simulink model "mLarge_MajorAdjust_3"  (R2019a)
settings: Solver=ode45  StartTime=0  StopTime=2000  FixedStep=0.001  RelTol=1e-5  AbsTol=1e-6
PostLoadFcn:
  | sldemo_fuelsys_data(bdroot,'initialize_data','orig','float');
model workspace (MAT data in the model file):
  PressEst = [0.806253176324 0.553142316929 0.37151500209 0.277667903103 0.220198954207 0.181288665766 0.153200000489 0.115431020872 0.0913067476324 0.0746519188607 0.0625231108324 0.0533383634277 ... (306 elements, 18x17)]
  PressVect = [0.05 0.1 0.15 0.2 0.25 0.3 0.35 0.4 0.45 0.5 0.55 0.6 0.65 0.7 0.75 0.8 0.85 0.9 0.95]
  PumpCon = [-0.0556348 -0.0022828 0.0256932 0.0435188 0.0562692 0.0661194857143 0.0741572 0.08697 0.0972452 0.106070342857 0.1139892 0.121303866667 ... (342 elements, 18x19)]
  RampRateKiX = [100 200 300 400 500 600]
  RampRateKiY = [0 0.2 0.4 0.6 0.8 1]
  RampRateKiZ = [0.012  0.024  0.036  0.048  0.06  0.072; 0.024  0.048  0.072  0.096  0.12  0.144; 0.036  0.072  0.108  0.144  0.18  0.216; 0.048  0.096  0.144  0.192  0.24  0.288; 0.06  0.12  0.18  0.24  0.3  0.36; 0.072  0.144  0.216  0.288  0.36  0.432]
  SpeedEst = [471.837839721 550.80940091 777.559313277 1080.9243499 1418.36795322 1769.7468768 2125.37309264 2480.20345067 2831.37796793 3177.14006959 3516.32917143 4064.90417867 ... (323 elements, 17x19)]
  SpeedVect = [50 75 100 125 150 175 200 250 300 350 400 450 500 600 700 800 900 1000]
  ThrotEst = [0 0 0 0 0 0 0 0 0 0 0 0 ... (342 elements, 18x19)]
  ThrotVect = [0 3 6 9 12 15 18 21 24 27 30 35 46 57 68 79 90]
  ego_sw = 1
  engine_speed = 300
  hys = 25
  map_sw = 1
  max_ego = 1.2
  max_press = 0.95
  max_speed = 628
  max_throt = 90
  min_press = 0.05
  min_speed = 50
  min_throt = 3
  speed_sw = 1
  st_range = 0.0001
  throttle_sw = 1
  zero_thresh = 250
undefined symbols (not defined in the file): DiscIntNeverNeededParam, sld_FuelModes, sldvsubsys
libraries: simulink x16, simulink_extras x4
(part 1 of 3)
CloseFcn:
  | clear EngSensors u8En* s16En* sldemo_fuelsys_output
Description:
  | This is a model of a fuel control system where Stateflow(R) is used to handle the fault management of the system.
  | The system contains four separate sensors: a throttle sensor, a speed sensor, an oxygen sensor, and a pressure sensor.
  | Each of these sensors is represented by a parallel state in Stateflow.  Each parallel state contains two substates, a
  | normal state and a failed state (the exception being the oxygen sensor, which also contains a warmup state).
  | 
  | If any of the sensor readings is outside an acceptable range, then a fault is registered in Stateflow, and the
  | substate of the corresponding subsystem transitions to the failed state.  If a subsystem recovers, it can
  | transition back to the normal state.  The number of failures in the system at any given time is represented
  | in the Fail parallel state.
  | 
  | The last parallel state in the Stateflow chart is called Fueling_Mode.  This state regulates the oxygen to
  | fuel mixture ratio.  If a failure is detected, then the oxygen to fuel ratio is increased.  If multiple failures
  | are detected, then the fuel system is disabled until there are no longer multiple failures in the system.
settings Model: ModifiedByFormat=The MathWorks Inc.  ExtModeTrigMode=oneshot  ExtModeArmWhenConnect=off  ExtModeAutoUpdateStatusClock=off  Creator=The MathWorks, Inc.  LastModifiedBy=The MathWorks Inc.
settings SolverCC: AutoScaleAbsTol=off
settings DataIOCC: SaveFormat=StructureWithTime  SaveOutput=off  SaveTime=off  ReturnWorkspaceOutputs=off  SignalLoggingName=sldemo_fuelsys_output
settings OptimizationCC: DefaultParameterBehavior=Inlined  UseDivisionForNetSlopeComputation=UseDivisionForReciprocalsOfIntegersOnly  InlineInvariantSignals=on  EnhancedBackFolding=on  StrengthReduction=on  BooleansAsBitfields=on  PassReuseOutputArgsAs=Individual arguments  ExpressionDepthLimit=2147483647  ZeroExternalMemoryAtStartup=off  ZeroInternalMemoryAtStartup=off  NoFixptDivByZeroProtection=on  EfficientFloat2IntCast=on  LifeSpan=1
settings DebuggingCC: SignalInfNanChecking=error  SaveWithParameterizedLinksMsg=none  UnderspecifiedInitializationDetection=Classic  CheckExecutionContextPreStartOutputMsg=on  CheckExecutionContextRuntimeOutputMsg=on  IntegerOverflowMsg=none  ParameterDowncastMsg=warning  ParameterOverflowMsg=none  ParameterPrecisionLossMsg=none  UnderSpecifiedDataTypeMsg=warning  FcnCallInpInsideContextMsg=warning  UniqueDataStoreMsg=error  BusObjectLabelMismatch=error  AllowSymbolicDim=off  StateNameClashWarn=warning  StrictBusMsg=ErrorOnBusTreatedAsVector  SFUnexpectedBacktrackingDiag=warning  SFNoUnconditionalDefaultTransitionDiag=warning  SFExecutionAtInitializationDiag=none  IntegerSaturationMsg=none
settings HardwareCC: ProdBitPerPointer=32  ProdBitPerSizeT=32  ProdBitPerPtrDiffT=32  ProdLargestAtomicFloat=None  ProdWordSize=32  ProdHWDeviceType=Specified
settings ModelReferenceCC: PropagateSignalLabelsOutOfModel=off
settings SFSimCC: SimUseLocalCustomCode=off  SimParseCustomCode=off  MATLABDynamicMemAlloc=off
settings RTWCC: SystemTargetFile=ert.tlc  TemplateMakefile=ert_default_tmf  Description=Real-Time Workshop Embedded Coder  GenerateReport=on  RTWVerbose=off  RTWUseLocalCustomCode=off  IncludeHyperlinkInReport=on  LaunchReport=on  GenerateTraceInfo=on  GenerateTraceReport=on  GenerateTraceReportSl=on  GenerateTraceReportSf=on  GenerateTraceReportEml=on
settings CodeAppCC: ForceParamTrailComments=on  IgnoreCustomStorageClasses=off  IgnoreTestpoints=on  SimulinkDataObjDesc=on  SFDataObjDesc=on  CustomSymbolStrGlobalVar=rt$N$M  CustomSymbolStrType=$N$M  CustomSymbolStrFcn=$N$M$F  CustomSymbolStrModelFcn=$N  CustomSymbolStrMacro=$N$M  InsertBlockDesc=on  StateflowObjectComments=on  InternalIdentifier=Classic  ReqsInCode=on
settings ERTTargetCC: MultiwordLength=2048  GenerateSampleERTMain=on  IncludeMdlTerminateFcn=off  SupportAbsoluteTime=off  SupportNonFinite=off  SupportComplex=off  InlinedParameterPlacement=NonHierarchical  ERTCustomFileTemplate=example_file_process.tlc  ConvertIfToSwitch=off  SuppressUnreachableDefaultCases=off
settings ConfigComp: CovScope=Subsystem  CovPath=/fuel_rate_control/control_logic  CovMetricSettings=dw  CovHtmlReporting=on  CovSaveCumulativeToWorkspaceVar=on  CovSaveSingleToWorkspaceVar=on  CovShowResultsExplorer=off  CovExternalEMLEnable=off  CovSFcnEnable=off

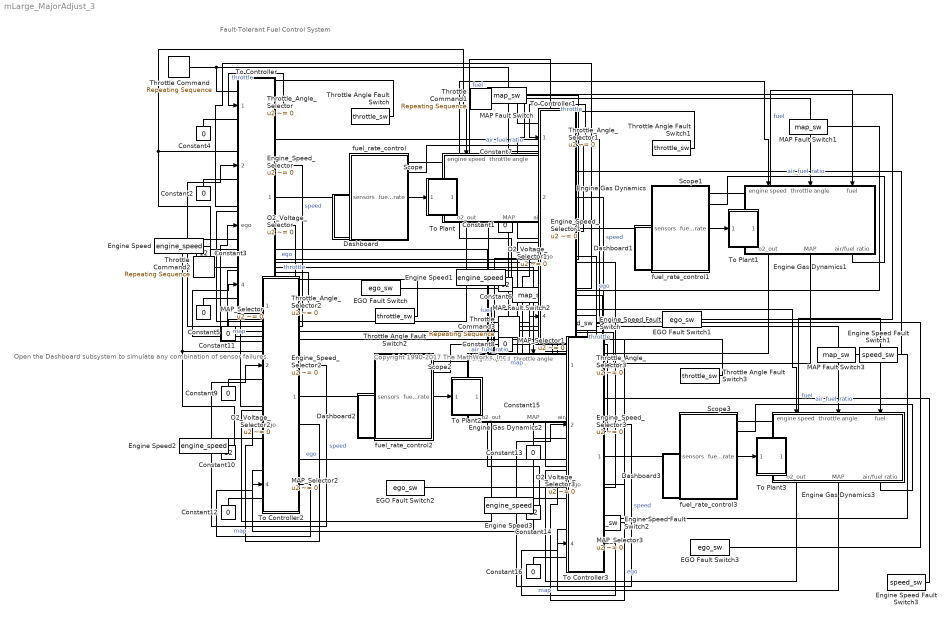
== system mLarge_MajorAdjust_3 ==
  note: Fault-Tolerant Fuel Control System
  note: Copyright 1990-2017 The MathWorks, Inc.
  note: Open the Dashboard subsystem to simulate any combination of sensor failures.
  Constant{1..2,4..5,7..9,11..13,15..16} (12 alike) : Constant  Value=0
  Constant{3,6,10,14} (4 alike) : Constant  Value=12
  Dashboard : Subsystem
  Dashboard1 : Subsystem
  Dashboard2 : Subsystem
  Dashboard3 : Subsystem
  EGO Fault Switch{,1..3} (4 alike) : Constant  Value=ego_sw
  Engine Gas Dynamics : Subsystem
  Engine Gas Dynamics1 : Subsystem
  Engine Gas Dynamics2 : Subsystem
  Engine Gas Dynamics3 : Subsystem
  Engine Speed{,1..3} (4 alike) : Constant  Value=engine_speed  SampleTime=[0,1]
  Engine Speed Fault Switch{,1..3} (4 alike) : Constant  Value=speed_sw
  Engine_Speed_Selector{,1..3} (4 alike) : Switch  Criteria=u2 ~= 0  Threshold=1
  MAP Fault Switch{,1..3} (4 alike) : Constant  Value=map_sw
  MAP_Selector{,1..3} (4 alike) : Switch  Criteria=u2 ~= 0  Threshold=1
  O2_Voltage_Selector{,1..3} (4 alike) : Switch  Criteria=u2 ~= 0  Threshold=1
  Scope{,1..3} (4 alike) : Scope  NumInputPorts=2
  Throttle Command{,1..3} (4 alike) : simulink/Sources/Repeating Sequence  rep_seq_t=[0 2 4]  rep_seq_y=[10 20 10]
  Throttle Angle Fault Switch{,1..3} (4 alike) : Constant  Value=throttle_sw
  Throttle_Angle_Selector{,1..3} (4 alike) : Switch  Criteria=u2 ~= 0  Threshold=1
  To Controller : Subsystem
      mask Display: fprintf('Convert')
  To Controller1 : Subsystem
      mask Display: fprintf('Convert')
  To Controller2 : Subsystem
      mask Display: fprintf('Convert')
  To Controller3 : Subsystem
      mask Display: fprintf('Convert')
  To Plant : Subsystem
      mask Display: fprintf('Convert')
  To Plant1 : Subsystem
      mask Display: fprintf('Convert')
  To Plant2 : Subsystem
      mask Display: fprintf('Convert')
  To Plant3 : Subsystem
      mask Display: fprintf('Convert')
  fuel_rate_control : Subsystem  Tag=FuelRateControl  TreatAsAtomicUnit=on
  fuel_rate_control1 : Subsystem  Tag=FuelRateControl  TreatAsAtomicUnit=on
  fuel_rate_control2 : Subsystem  Tag=FuelRateControl  TreatAsAtomicUnit=on
  fuel_rate_control3 : Subsystem  Tag=FuelRateControl  TreatAsAtomicUnit=on
  wires:
  fuel_rate_control/1(fuel_rate) -> To Plant/1(In1)
  To Plant/1(Out1) -> Scope/1, Engine Gas Dynamics/3(fuel)  "fuel"
  To Controller/1(sensors) -> fuel_rate_control/1(sensors)
  Throttle_Angle_Selector/1 -> To Controller/1(throttle)  "throttle"
  Engine_Speed_Selector/1 -> To Controller/2(speed)  "speed"
  O2_Voltage_Selector/1 -> To Controller/3(ego)  "ego"
  MAP_Selector/1 -> To Controller/4(map)  "map"
  Constant4/1 -> Throttle_Angle_Selector/3
  Throttle Command/1 -> Throttle_Angle_Selector/1, Engine Gas Dynamics/2(throttle angle)
  Throttle Angle Fault Switch/1 -> Throttle_Angle_Selector/2
  Engine Speed Fault Switch/1 -> Engine_Speed_Selector/2
  Engine Speed/1 -> Engine_Speed_Selector/1, Engine Gas Dynamics/1(engine speed)
  Constant2/1 -> Engine_Speed_Selector/3
  Constant3/1 -> O2_Voltage_Selector/3
  Engine Gas Dynamics/1(o2_out) -> O2_Voltage_Selector/1
  EGO Fault Switch/1 -> O2_Voltage_Selector/2
  MAP Fault Switch/1 -> MAP_Selector/2
  Engine Gas Dynamics/2(MAP) -> MAP_Selector/1
  Constant5/1 -> MAP_Selector/3
  Engine Gas Dynamics/3(air/fuel ratio) -> Scope/2  "air_fuel_ratio"
  Engine Speed Fault Switch1/1 -> Engine_Speed_Selector1/2
  fuel_rate_control1/1(fuel_rate) -> To Plant1/1(In1)
  O2_Voltage_Selector1/1 -> To Controller1/3(ego)  "ego"
  Engine Gas Dynamics1/3(air/fuel ratio) -> Scope1/2  "air_fuel_ratio"
  Throttle Angle Fault Switch1/1 -> Throttle_Angle_Selector1/2
  To Controller1/1(sensors) -> fuel_rate_control1/1(sensors)
  To Plant1/1(Out1) -> Scope1/1, Engine Gas Dynamics1/3(fuel)  "fuel"
  Engine_Speed_Selector1/1 -> To Controller1/2(speed)  "speed"
  Engine Gas Dynamics1/2(MAP) -> MAP_Selector1/1
  Constant8/1 -> MAP_Selector1/3
  MAP_Selector1/1 -> To Controller1/4(map)  "map"
  Constant7/1 -> Throttle_Angle_Selector1/3
  Throttle Command1/1 -> Throttle_Angle_Selector1/1, Engine Gas Dynamics1/2(throttle angle)
  Constant6/1 -> O2_Voltage_Selector1/3
  Engine Speed1/1 -> Engine_Speed_Selector1/1, Engine Gas Dynamics1/1(engine speed)
  Throttle_Angle_Selector1/1 -> To Controller1/1(throttle)  "throttle"
  MAP Fault Switch1/1 -> MAP_Selector1/2
  Engine Gas Dynamics1/1(o2_out) -> O2_Voltage_Selector1/1
  EGO Fault Switch1/1 -> O2_Voltage_Selector1/2
  Constant1/1 -> Engine_Speed_Selector1/3
  Engine Speed Fault Switch2/1 -> Engine_Speed_Selector2/2
  fuel_rate_control2/1(fuel_rate) -> To Plant2/1(In1)
  O2_Voltage_Selector2/1 -> To Controller2/3(ego)  "ego"
  Engine Gas Dynamics2/3(air/fuel ratio) -> Scope2/2  "air_fuel_ratio"
  Throttle Angle Fault Switch2/1 -> Throttle_Angle_Selector2/2
  To Controller2/1(sensors) -> fuel_rate_control2/1(sensors)
  To Plant2/1(Out1) -> Scope2/1, Engine Gas Dynamics2/3(fuel)  "fuel"
  Engine_Speed_Selector2/1 -> To Controller2/2(speed)  "speed"
  Engine Gas Dynamics2/2(MAP) -> MAP_Selector2/1
  Constant12/1 -> MAP_Selector2/3
  MAP_Selector2/1 -> To Controller2/4(map)  "map"
  Constant11/1 -> Throttle_Angle_Selector2/3
  Throttle Command2/1 -> Throttle_Angle_Selector2/1, Engine Gas Dynamics2/2(throttle angle)
  Constant10/1 -> O2_Voltage_Selector2/3
  Engine Speed2/1 -> Engine_Speed_Selector2/1, Engine Gas Dynamics2/1(engine speed)
  Throttle_Angle_Selector2/1 -> To Controller2/1(throttle)  "throttle"
  MAP Fault Switch2/1 -> MAP_Selector2/2
  Engine Gas Dynamics2/1(o2_out) -> O2_Voltage_Selector2/1
  EGO Fault Switch2/1 -> O2_Voltage_Selector2/2
  Constant9/1 -> Engine_Speed_Selector2/3
  Engine Speed Fault Switch3/1 -> Engine_Speed_Selector3/2
  fuel_rate_control3/1(fuel_rate) -> To Plant3/1(In1)
  O2_Voltage_Selector3/1 -> To Controller3/3(ego)  "ego"
  Engine Gas Dynamics3/3(air/fuel ratio) -> Scope3/2  "air_fuel_ratio"
  Throttle Angle Fault Switch3/1 -> Throttle_Angle_Selector3/2
  To Controller3/1(sensors) -> fuel_rate_control3/1(sensors)
  To Plant3/1(Out1) -> Scope3/1, Engine Gas Dynamics3/3(fuel)  "fuel"
  Engine_Speed_Selector3/1 -> To Controller3/2(speed)  "speed"
  Engine Gas Dynamics3/2(MAP) -> MAP_Selector3/1
  Constant16/1 -> MAP_Selector3/3
  MAP_Selector3/1 -> To Controller3/4(map)  "map"
  Constant15/1 -> Throttle_Angle_Selector3/3
  Throttle Command3/1 -> Throttle_Angle_Selector3/1, Engine Gas Dynamics3/2(throttle angle)
  Constant14/1 -> O2_Voltage_Selector3/3
  Engine Speed3/1 -> Engine_Speed_Selector3/1, Engine Gas Dynamics3/1(engine speed)
  Throttle_Angle_Selector3/1 -> To Controller3/1(throttle)  "throttle"
  MAP Fault Switch3/1 -> MAP_Selector3/2
  Engine Gas Dynamics3/1(o2_out) -> O2_Voltage_Selector3/1
  EGO Fault Switch3/1 -> O2_Voltage_Selector3/2
  Constant13/1 -> Engine_Speed_Selector3/3

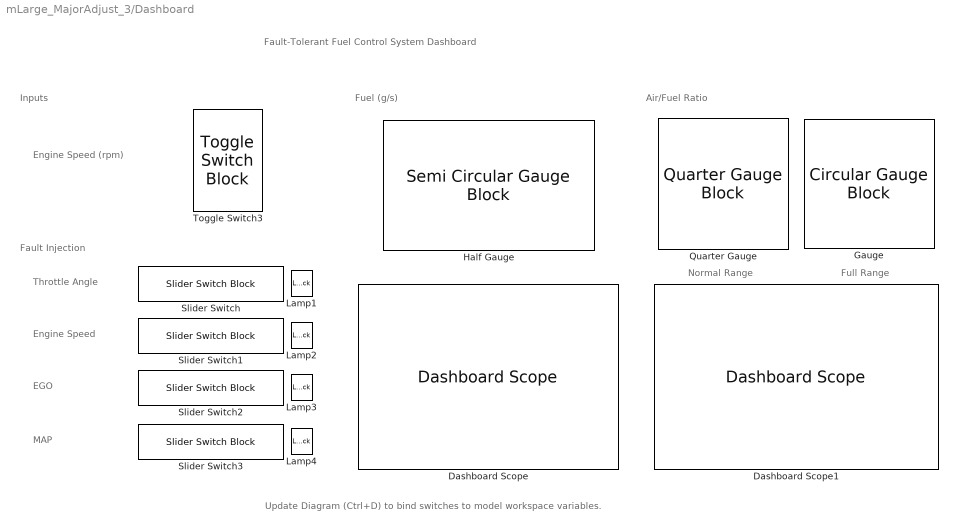
== system mLarge_MajorAdjust_3/Dashboard ==
  note: Inputs
  note: Fault Injection
  note: Air/Fuel Ratio
  note: Fuel (g/s)
  note: Throttle Angle
  note: Engine Speed
  note: EGO
  note: Fault-Tolerant Fuel Control System Dashboard
  note: MAP
  note: Engine Speed (rpm)
  note: Normal Range
  note: Full Range
  note: Update Diagram (Ctrl+D) to bind switches to model workspace variables.
  Dashboard Scope : DashboardScope  WebBlockId=348  TimeSpan=500  Ymin=0  LegendPosition=Hide  ScaleAtStop=off
  Dashboard Scope1 : DashboardScope  WebBlockId=349  TimeSpan=500  Ymin=0  Ymax=400  LegendPosition=Hide  ScaleAtStop=off
  Gauge : CircularGaugeBlock  WebBlockId=346  LabelPosition=Hide  ScaleMax=400
  Half Gauge : SemiCircularGaugeBlock  WebBlockId=347  LabelPosition=Hide  ScaleMax=3
  Lamp1 : LampBlock  WebBlockId=337  LabelPosition=Hide
  Lamp2 : LampBlock  WebBlockId=338  LabelPosition=Hide
  Lamp3 : LampBlock  WebBlockId=343  LabelPosition=Hide
  Lamp4 : LampBlock  WebBlockId=339  LabelPosition=Hide
  Quarter Gauge : QuarterGaugeBlock  WebBlockId=345  LabelPosition=Hide  ScaleMax=20
  Slider Switch : SliderSwitchBlock  WebBlockId=341  LabelPosition=Hide
      settings: Values={{'NORMAL', 'FAIL'}, [1 0]}
  Slider Switch1 : SliderSwitchBlock  WebBlockId=342  LabelPosition=Hide
      settings: Values={{'NORMAL', 'FAIL'}, [1 0]}
  Slider Switch2 : SliderSwitchBlock  WebBlockId=344  LabelPosition=Hide
      settings: Values={{'NORMAL', 'FAIL'}, [1 0]}
  Slider Switch3 : SliderSwitchBlock  WebBlockId=340  LabelPosition=Hide
      settings: Values={{'NORMAL', 'FAIL'}, [1 0]}
  Toggle Switch3 : ToggleSwitchBlock  WebBlockId=336  LabelPosition=Hide
      settings: Values={{'700', '300'}, [700 300]}

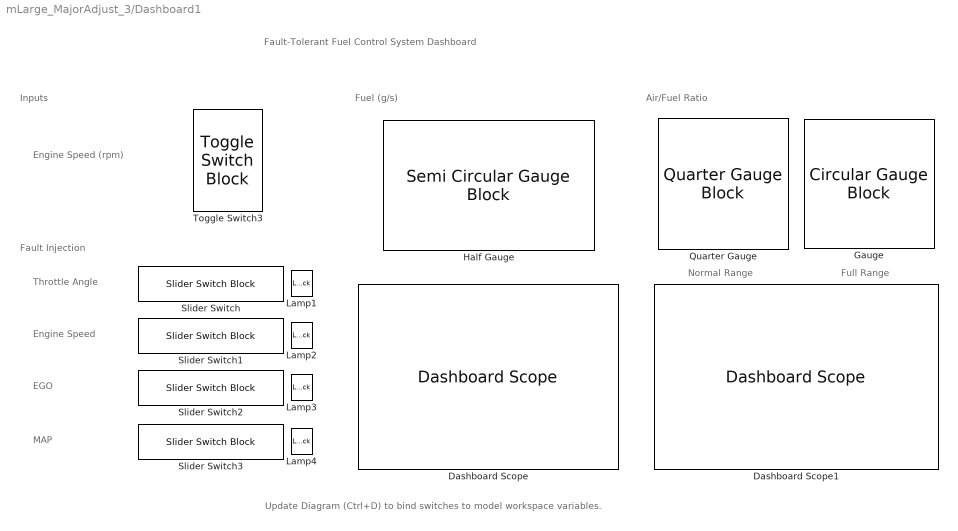
== system mLarge_MajorAdjust_3/Dashboard1 ==
  note: Inputs
  note: Fault Injection
  note: Air/Fuel Ratio
  note: Fuel (g/s)
  note: Throttle Angle
  note: Engine Speed
  note: EGO
  note: Fault-Tolerant Fuel Control System Dashboard
  note: MAP
  note: Engine Speed (rpm)
  note: Normal Range
  note: Full Range
  note: Update Diagram (Ctrl+D) to bind switches to model workspace variables.
  Dashboard Scope : DashboardScope  WebBlockId=355  TimeSpan=500  Ymin=0  LegendPosition=Hide  ScaleAtStop=off
  Dashboard Scope1 : DashboardScope  WebBlockId=356  TimeSpan=500  Ymin=0  Ymax=400  LegendPosition=Hide  ScaleAtStop=off
  Gauge : CircularGaugeBlock  WebBlockId=357  LabelPosition=Hide  ScaleMax=400
  Half Gauge : SemiCircularGaugeBlock  WebBlockId=358  LabelPosition=Hide  ScaleMax=3
  Lamp1 : LampBlock  WebBlockId=359  LabelPosition=Hide
  Lamp2 : LampBlock  WebBlockId=360  LabelPosition=Hide
  Lamp3 : LampBlock  WebBlockId=361  LabelPosition=Hide
  Lamp4 : LampBlock  WebBlockId=362  LabelPosition=Hide
  Quarter Gauge : QuarterGaugeBlock  WebBlockId=363  LabelPosition=Hide  ScaleMax=20
  Slider Switch : SliderSwitchBlock  WebBlockId=364  LabelPosition=Hide
      settings: Values={{'NORMAL', 'FAIL'}, [1 0]}
  Slider Switch1 : SliderSwitchBlock  WebBlockId=365  LabelPosition=Hide
      settings: Values={{'NORMAL', 'FAIL'}, [1 0]}
  Slider Switch2 : SliderSwitchBlock  WebBlockId=366  LabelPosition=Hide
      settings: Values={{'NORMAL', 'FAIL'}, [1 0]}
  Slider Switch3 : SliderSwitchBlock  WebBlockId=367  LabelPosition=Hide
      settings: Values={{'NORMAL', 'FAIL'}, [1 0]}
  Toggle Switch3 : ToggleSwitchBlock  WebBlockId=368  LabelPosition=Hide
      settings: Values={{'700', '300'}, [700 300]}

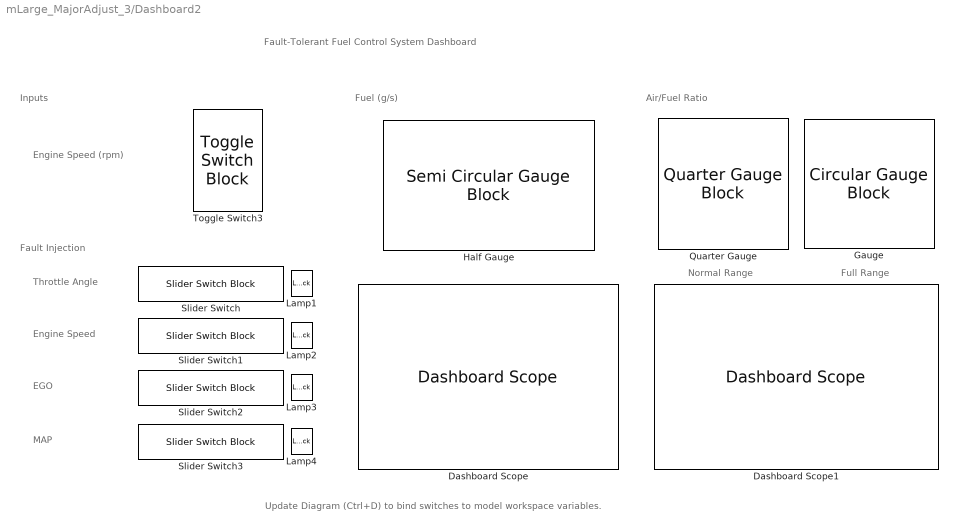
== system mLarge_MajorAdjust_3/Dashboard2 ==
  note: Inputs
  note: Fault Injection
  note: Air/Fuel Ratio
  note: Fuel (g/s)
  note: Throttle Angle
  note: Engine Speed
  note: EGO
  note: Fault-Tolerant Fuel Control System Dashboard
  note: MAP
  note: Engine Speed (rpm)
  note: Normal Range
  note: Full Range
  note: Update Diagram (Ctrl+D) to bind switches to model workspace variables.
  Dashboard Scope : DashboardScope  WebBlockId=551  TimeSpan=500  Ymin=0  LegendPosition=Hide  ScaleAtStop=off
  Dashboard Scope1 : DashboardScope  WebBlockId=552  TimeSpan=500  Ymin=0  Ymax=400  LegendPosition=Hide  ScaleAtStop=off
  Gauge : CircularGaugeBlock  WebBlockId=553  LabelPosition=Hide  ScaleMax=400
  Half Gauge : SemiCircularGaugeBlock  WebBlockId=554  LabelPosition=Hide  ScaleMax=3
  Lamp1 : LampBlock  WebBlockId=555  LabelPosition=Hide
  Lamp2 : LampBlock  WebBlockId=556  LabelPosition=Hide
  Lamp3 : LampBlock  WebBlockId=557  LabelPosition=Hide
  Lamp4 : LampBlock  WebBlockId=558  LabelPosition=Hide
  Quarter Gauge : QuarterGaugeBlock  WebBlockId=559  LabelPosition=Hide  ScaleMax=20
  Slider Switch : SliderSwitchBlock  WebBlockId=560  LabelPosition=Hide
      settings: Values={{'NORMAL', 'FAIL'}, [1 0]}
  Slider Switch1 : SliderSwitchBlock  WebBlockId=561  LabelPosition=Hide
      settings: Values={{'NORMAL', 'FAIL'}, [1 0]}
  Slider Switch2 : SliderSwitchBlock  WebBlockId=562  LabelPosition=Hide
      settings: Values={{'NORMAL', 'FAIL'}, [1 0]}
  Slider Switch3 : SliderSwitchBlock  WebBlockId=563  LabelPosition=Hide
      settings: Values={{'NORMAL', 'FAIL'}, [1 0]}
  Toggle Switch3 : ToggleSwitchBlock  WebBlockId=564  LabelPosition=Hide
      settings: Values={{'700', '300'}, [700 300]}

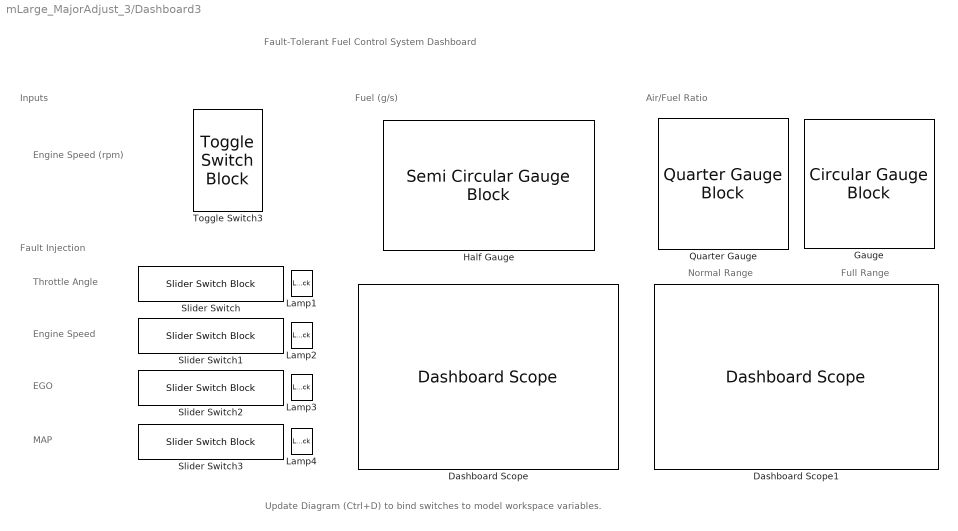
== system mLarge_MajorAdjust_3/Dashboard3 ==
  note: Inputs
  note: Fault Injection
  note: Air/Fuel Ratio
  note: Fuel (g/s)
  note: Throttle Angle
  note: Engine Speed
  note: EGO
  note: Fault-Tolerant Fuel Control System Dashboard
  note: MAP
  note: Engine Speed (rpm)
  note: Normal Range
  note: Full Range
  note: Update Diagram (Ctrl+D) to bind switches to model workspace variables.
  Dashboard Scope : DashboardScope  WebBlockId=747  TimeSpan=500  Ymin=0  LegendPosition=Hide  ScaleAtStop=off
  Dashboard Scope1 : DashboardScope  WebBlockId=748  TimeSpan=500  Ymin=0  Ymax=400  LegendPosition=Hide  ScaleAtStop=off
  Gauge : CircularGaugeBlock  WebBlockId=749  LabelPosition=Hide  ScaleMax=400
  Half Gauge : SemiCircularGaugeBlock  WebBlockId=750  LabelPosition=Hide  ScaleMax=3
  Lamp1 : LampBlock  WebBlockId=751  LabelPosition=Hide
  Lamp2 : LampBlock  WebBlockId=752  LabelPosition=Hide
  Lamp3 : LampBlock  WebBlockId=753  LabelPosition=Hide
  Lamp4 : LampBlock  WebBlockId=754  LabelPosition=Hide
  Quarter Gauge : QuarterGaugeBlock  WebBlockId=755  LabelPosition=Hide  ScaleMax=20
  Slider Switch : SliderSwitchBlock  WebBlockId=756  LabelPosition=Hide
      settings: Values={{'NORMAL', 'FAIL'}, [1 0]}
  Slider Switch1 : SliderSwitchBlock  WebBlockId=757  LabelPosition=Hide
      settings: Values={{'NORMAL', 'FAIL'}, [1 0]}
  Slider Switch2 : SliderSwitchBlock  WebBlockId=758  LabelPosition=Hide
      settings: Values={{'NORMAL', 'FAIL'}, [1 0]}
  Slider Switch3 : SliderSwitchBlock  WebBlockId=759  LabelPosition=Hide
      settings: Values={{'NORMAL', 'FAIL'}, [1 0]}
  Toggle Switch3 : ToggleSwitchBlock  WebBlockId=760  LabelPosition=Hide
      settings: Values={{'700', '300'}, [700 300]}

== system mLarge_MajorAdjust_3/Engine Gas Dynamics ==
  engine speed : Inport  Unit=rad/s
  throttle angle : Inport  Port=2  Unit=deg
  fuel : Inport  Port=3  Unit=g/s
  Mixing & Combustion : Subsystem
  Throttle & Manifold : Subsystem
  o2_out : Outport  Unit=V
  MAP : Outport  Port=2  Unit=bar
  air/fuel ratio : Outport  Port=3  Unit=1
  wires:
  Throttle & Manifold/1(Mass Airflow Rate) -> Mixing & Combustion/2(air flow)
  fuel/1 -> Mixing & Combustion/1(fuel rate)
  engine speed/1 -> Throttle & Manifold/1("Engine Speed, N")
  throttle angle/1 -> Throttle & Manifold/2(Throttle Ang.)
  Mixing & Combustion/2(air/fuel ratio) -> air/fuel ratio/1
  Throttle & Manifold/2(MAP (bar)) -> MAP/1
  Mixing & Combustion/1(o2_out) -> o2_out/1

== system mLarge_MajorAdjust_3/Engine Gas Dynamics1 ==
  engine speed : Inport  Unit=rad/s
  throttle angle : Inport  Port=2  Unit=deg
  fuel : Inport  Port=3  Unit=g/s
  Mixing & Combustion : Subsystem
  Throttle & Manifold : Subsystem
  o2_out : Outport  Unit=V
  MAP : Outport  Port=2  Unit=bar
  air/fuel ratio : Outport  Port=3  Unit=1
  wires:
  Throttle & Manifold/1(Mass Airflow Rate) -> Mixing & Combustion/2(air flow)
  fuel/1 -> Mixing & Combustion/1(fuel rate)
  engine speed/1 -> Throttle & Manifold/1("Engine Speed, N")
  throttle angle/1 -> Throttle & Manifold/2(Throttle Ang.)
  Mixing & Combustion/2(air/fuel ratio) -> air/fuel ratio/1
  Throttle & Manifold/2(MAP (bar)) -> MAP/1
  Mixing & Combustion/1(o2_out) -> o2_out/1

== system mLarge_MajorAdjust_3/Engine Gas Dynamics2 ==
  engine speed : Inport  Unit=rad/s
  throttle angle : Inport  Port=2  Unit=deg
  fuel : Inport  Port=3  Unit=g/s
  Mixing & Combustion : Subsystem
  Throttle & Manifold : Subsystem
  o2_out : Outport  Unit=V
  MAP : Outport  Port=2  Unit=bar
  air/fuel ratio : Outport  Port=3  Unit=1
  wires:
  Throttle & Manifold/1(Mass Airflow Rate) -> Mixing & Combustion/2(air flow)
  fuel/1 -> Mixing & Combustion/1(fuel rate)
  engine speed/1 -> Throttle & Manifold/1("Engine Speed, N")
  throttle angle/1 -> Throttle & Manifold/2(Throttle Ang.)
  Mixing & Combustion/2(air/fuel ratio) -> air/fuel ratio/1
  Throttle & Manifold/2(MAP (bar)) -> MAP/1
  Mixing & Combustion/1(o2_out) -> o2_out/1

== system mLarge_MajorAdjust_3/Engine Gas Dynamics3 ==
  engine speed : Inport  Unit=rad/s
  throttle angle : Inport  Port=2  Unit=deg
  fuel : Inport  Port=3  Unit=g/s
  Mixing & Combustion : Subsystem
  Throttle & Manifold : Subsystem
  o2_out : Outport  Unit=V
  MAP : Outport  Port=2  Unit=bar
  air/fuel ratio : Outport  Port=3  Unit=1
  wires:
  Throttle & Manifold/1(Mass Airflow Rate) -> Mixing & Combustion/2(air flow)
  fuel/1 -> Mixing & Combustion/1(fuel rate)
  engine speed/1 -> Throttle & Manifold/1("Engine Speed, N")
  throttle angle/1 -> Throttle & Manifold/2(Throttle Ang.)
  Mixing & Combustion/2(air/fuel ratio) -> air/fuel ratio/1
  Throttle & Manifold/2(MAP (bar)) -> MAP/1
  Mixing & Combustion/1(o2_out) -> o2_out/1

== system mLarge_MajorAdjust_3/To Controller ==
  note: This system:
      | - Packs individual sensors into a EngSensors bus signal
      | - Permits bus elements data types to change
      | - Converts signals from continuous to discrete time
  throttle : Inport
  speed : Inport  Port=2
  ego : Inport  Port=3
  map : Inport  Port=4
  Bus Creator : BusCreator  Inputs=4  OutDataTypeStr=Bus: EngSensors  NonVirtualBus=on
  DTC{1..4} (4 alike) : DataTypeConversion  SampleTime=[0 1]
  Rate Transition : RateTransition  OutPortSampleTime=0.01
  Sensor Info : simulink/Model-Wide Utilities/DocBlock  DocumentType=Text
      content=|
      | Measurement Descriptions
      | ========================
      |
      | Throttle Angle (degrees):
      | min=3, max=90, precision=0.1
      |
      | Engine Speed (radians/sec.):
      | min=0, max=620, precision=.1
      |
      | Ego Sensor (volts):
      | min=0, max=12, precision=.05
      |
      | Manifold Pressure (bar):
      | min=0.001, max=1, precision=.001
  sensors : Outport
  wires:
  throttle/1 -> DTC1/1
  DTC1/1 -> Bus Creator/1  "throttle"
  speed/1 -> DTC2/1
  DTC2/1 -> Bus Creator/2  "speed"
  ego/1 -> DTC3/1
  DTC3/1 -> Bus Creator/3  "ego"
  map/1 -> DTC4/1
  DTC4/1 -> Bus Creator/4  "map"
  Bus Creator/1 -> Rate Transition/1
  Rate Transition/1 -> sensors/1

== system mLarge_MajorAdjust_3/To Controller1 ==
  note: This system:
      | - Packs individual sensors into a EngSensors bus signal
      | - Permits bus elements data types to change
      | - Converts signals from continuous to discrete time
  throttle : Inport
  speed : Inport  Port=2
  ego : Inport  Port=3
  map : Inport  Port=4
  Bus Creator : BusCreator  Inputs=4  OutDataTypeStr=Bus: EngSensors  NonVirtualBus=on
  DTC{1..4} (4 alike) : DataTypeConversion  SampleTime=[0 1]
  Rate Transition : RateTransition  OutPortSampleTime=0.01
  Sensor Info : simulink/Model-Wide Utilities/DocBlock  DocumentType=Text
      content=|
      | Measurement Descriptions
      | ========================
      |
      | Throttle Angle (degrees):
      | min=3, max=90, precision=0.1
      |
      | Engine Speed (radians/sec.):
      | min=0, max=620, precision=.1
      |
      | Ego Sensor (volts):
      | min=0, max=12, precision=.05
      |
      | Manifold Pressure (bar):
      | min=0.001, max=1, precision=.001
  sensors : Outport
  wires:
  throttle/1 -> DTC1/1
  DTC1/1 -> Bus Creator/1  "throttle"
  speed/1 -> DTC2/1
  DTC2/1 -> Bus Creator/2  "speed"
  ego/1 -> DTC3/1
  DTC3/1 -> Bus Creator/3  "ego"
  map/1 -> DTC4/1
  DTC4/1 -> Bus Creator/4  "map"
  Bus Creator/1 -> Rate Transition/1
  Rate Transition/1 -> sensors/1

== system mLarge_MajorAdjust_3/To Controller2 ==
  note: This system:
      | - Packs individual sensors into a EngSensors bus signal
      | - Permits bus elements data types to change
      | - Converts signals from continuous to discrete time
  throttle : Inport
  speed : Inport  Port=2
  ego : Inport  Port=3
  map : Inport  Port=4
  Bus Creator : BusCreator  Inputs=4  OutDataTypeStr=Bus: EngSensors  NonVirtualBus=on
  DTC{1..4} (4 alike) : DataTypeConversion  SampleTime=[0 1]
  Rate Transition : RateTransition  OutPortSampleTime=0.01
  Sensor Info : simulink/Model-Wide Utilities/DocBlock  DocumentType=Text
      content=|
      | Measurement Descriptions
      | ========================
      |
      | Throttle Angle (degrees):
      | min=3, max=90, precision=0.1
      |
      | Engine Speed (radians/sec.):
      | min=0, max=620, precision=.1
      |
      | Ego Sensor (volts):
      | min=0, max=12, precision=.05
      |
      | Manifold Pressure (bar):
      | min=0.001, max=1, precision=.001
  sensors : Outport
  wires:
  throttle/1 -> DTC1/1
  DTC1/1 -> Bus Creator/1  "throttle"
  speed/1 -> DTC2/1
  DTC2/1 -> Bus Creator/2  "speed"
  ego/1 -> DTC3/1
  DTC3/1 -> Bus Creator/3  "ego"
  map/1 -> DTC4/1
  DTC4/1 -> Bus Creator/4  "map"
  Bus Creator/1 -> Rate Transition/1
  Rate Transition/1 -> sensors/1

== system mLarge_MajorAdjust_3/To Controller3 ==
  note: This system:
      | - Packs individual sensors into a EngSensors bus signal
      | - Permits bus elements data types to change
      | - Converts signals from continuous to discrete time
  throttle : Inport
  speed : Inport  Port=2
  ego : Inport  Port=3
  map : Inport  Port=4
  Bus Creator : BusCreator  Inputs=4  OutDataTypeStr=Bus: EngSensors  NonVirtualBus=on
  DTC{1..4} (4 alike) : DataTypeConversion  SampleTime=[0 1]
  Rate Transition : RateTransition  OutPortSampleTime=0.01
  Sensor Info : simulink/Model-Wide Utilities/DocBlock  DocumentType=Text
      content=|
      | Measurement Descriptions
      | ========================
      |
      | Throttle Angle (degrees):
      | min=3, max=90, precision=0.1
      |
      | Engine Speed (radians/sec.):
      | min=0, max=620, precision=.1
      |
      | Ego Sensor (volts):
      | min=0, max=12, precision=.05
      |
      | Manifold Pressure (bar):
      | min=0.001, max=1, precision=.001
  sensors : Outport
  wires:
  throttle/1 -> DTC1/1
  DTC1/1 -> Bus Creator/1  "throttle"
  speed/1 -> DTC2/1
  DTC2/1 -> Bus Creator/2  "speed"
  ego/1 -> DTC3/1
  DTC3/1 -> Bus Creator/3  "ego"
  map/1 -> DTC4/1
  DTC4/1 -> Bus Creator/4  "map"
  Bus Creator/1 -> Rate Transition/1
  Rate Transition/1 -> sensors/1

== system mLarge_MajorAdjust_3/To Plant ==
  note: This system:
      | - Permits upstream signal data type to change
      | - Converts signals from discrete to continuous time
  In1 : Inport
  DTC5 : DataTypeConversion
  Rate Transition1 : RateTransition  Integrity=off  InitialCondition=1.6  OutPortSampleTime=0
  Out1 : Outport
  wires:
  DTC5/1 -> Rate Transition1/1
  In1/1 -> DTC5/1
  Rate Transition1/1 -> Out1/1

== system mLarge_MajorAdjust_3/To Plant1 ==
  note: This system:
      | - Permits upstream signal data type to change
      | - Converts signals from discrete to continuous time
  In1 : Inport
  DTC5 : DataTypeConversion
  Rate Transition1 : RateTransition  Integrity=off  InitialCondition=1.6  OutPortSampleTime=0
  Out1 : Outport
  wires:
  DTC5/1 -> Rate Transition1/1
  In1/1 -> DTC5/1
  Rate Transition1/1 -> Out1/1

== system mLarge_MajorAdjust_3/To Plant2 ==
  note: This system:
      | - Permits upstream signal data type to change
      | - Converts signals from discrete to continuous time
  In1 : Inport
  DTC5 : DataTypeConversion
  Rate Transition1 : RateTransition  Integrity=off  InitialCondition=1.6  OutPortSampleTime=0
  Out1 : Outport
  wires:
  DTC5/1 -> Rate Transition1/1
  In1/1 -> DTC5/1
  Rate Transition1/1 -> Out1/1

== system mLarge_MajorAdjust_3/To Plant3 ==
  note: This system:
      | - Permits upstream signal data type to change
      | - Converts signals from discrete to continuous time
  In1 : Inport
  DTC5 : DataTypeConversion
  Rate Transition1 : RateTransition  Integrity=off  InitialCondition=1.6  OutPortSampleTime=0
  Out1 : Outport
  wires:
  DTC5/1 -> Rate Transition1/1
  In1/1 -> DTC5/1
  Rate Transition1/1 -> Out1/1

== system mLarge_MajorAdjust_3/fuel_rate_control ==
  note: Fuel Rate Control Subsystem
  sensors : Inport  OutDataTypeStr=Bus: EngSensors
  Bus Selector1 : BusSelector  OutputSignals=speed
  airflow_calc : Subsystem
  control_logic : Stateflow chart  Description=Stateflow diagram to determine control system operating mode  TreatAsAtomicUnit=on
  fuel_calc : Subsystem
  validate_sample_time : Subsystem  Tag=VerificationSubsystem  DisableCoverage=on  LoadFcn=sldvsubsys('check')  TreatAsAtomicUnit=on  SimViewingDevice=on  mask(VerificationSubsystem){}
      mask init:
      | sldvsubsys('maskInit');
      settings: CopyFcn=sldvsubsys('copy');  OpenFcn=open_system(gcb,'force');
      settings: PreSaveFcn=|
      | set_param(gcb,'SimViewingDevice','on');
      | sldvsubsys('check');
      mask Help: helpview(fullfile(docroot,'toolbox','sldv','sldv.map'),'verificationsubsystem')
      mask Display: image(imread('sldvicon_versubsys.png','BackGroundColor',[1 1 1]),'center');
  fuel_rate : Outport  Unit=g/s
  wires:
  fuel_calc/1(fuel_rate) -> fuel_rate/1
  airflow_calc/1(est_airflow) -> fuel_calc/1(est_airflow)
  sensors/1 -> control_logic/1(es_i), Bus Selector1/1
  control_logic/3(fuel_mode) -> airflow_calc/3(fuel_mode), fuel_calc/3(fuel_mode)
  control_logic/1(es_o) -> airflow_calc/1(sensors)
  control_logic/2(" O2_normal") -> airflow_calc/2(O2_normal)
  airflow_calc/2(fb_correction) -> fuel_calc/2(fb_correction)
  Bus Selector1/1 -> validate_sample_time/1(In1)  "<speed>"

== system mLarge_MajorAdjust_3/fuel_rate_control1 ==
  note: Fuel Rate Control Subsystem
  sensors : Inport  OutDataTypeStr=Bus: EngSensors
  Bus Selector1 : BusSelector  OutputSignals=speed
  airflow_calc : Subsystem
  control_logic : Stateflow chart  Description=Stateflow diagram to determine control system operating mode  TreatAsAtomicUnit=on
  fuel_calc : Subsystem
  validate_sample_time : Subsystem  Tag=VerificationSubsystem  DisableCoverage=on  LoadFcn=sldvsubsys('check')  TreatAsAtomicUnit=on  SimViewingDevice=on  mask(VerificationSubsystem){}
      mask init:
      | sldvsubsys('maskInit');
      settings: CopyFcn=sldvsubsys('copy');  OpenFcn=open_system(gcb,'force');
      settings: PreSaveFcn=|
      | set_param(gcb,'SimViewingDevice','on');
      | sldvsubsys('check');
      mask Help: helpview(fullfile(docroot,'toolbox','sldv','sldv.map'),'verificationsubsystem')
      mask Display: image(imread('sldvicon_versubsys.png','BackGroundColor',[1 1 1]),'center');
  fuel_rate : Outport  Unit=g/s
  wires:
  fuel_calc/1(fuel_rate) -> fuel_rate/1
  airflow_calc/1(est_airflow) -> fuel_calc/1(est_airflow)
  sensors/1 -> control_logic/1(es_i), Bus Selector1/1
  control_logic/3(fuel_mode) -> airflow_calc/3(fuel_mode), fuel_calc/3(fuel_mode)
  control_logic/1(es_o) -> airflow_calc/1(sensors)
  control_logic/2(" O2_normal") -> airflow_calc/2(O2_normal)
  airflow_calc/2(fb_correction) -> fuel_calc/2(fb_correction)
  Bus Selector1/1 -> validate_sample_time/1(In1)  "<speed>"

== system mLarge_MajorAdjust_3/fuel_rate_control2 ==
  note: Fuel Rate Control Subsystem
  sensors : Inport  OutDataTypeStr=Bus: EngSensors
  Bus Selector1 : BusSelector  OutputSignals=speed
  airflow_calc : Subsystem
  control_logic : Stateflow chart  Description=Stateflow diagram to determine control system operating mode  TreatAsAtomicUnit=on
  fuel_calc : Subsystem
  validate_sample_time : Subsystem  Tag=VerificationSubsystem  DisableCoverage=on  LoadFcn=sldvsubsys('check')  TreatAsAtomicUnit=on  SimViewingDevice=on  mask(VerificationSubsystem){}
      mask init:
      | sldvsubsys('maskInit');
      settings: CopyFcn=sldvsubsys('copy');  OpenFcn=open_system(gcb,'force');
      settings: PreSaveFcn=|
      | set_param(gcb,'SimViewingDevice','on');
      | sldvsubsys('check');
      mask Help: helpview(fullfile(docroot,'toolbox','sldv','sldv.map'),'verificationsubsystem')
      mask Display: image(imread('sldvicon_versubsys.png','BackGroundColor',[1 1 1]),'center');
  fuel_rate : Outport  Unit=g/s
  wires:
  fuel_calc/1(fuel_rate) -> fuel_rate/1
  airflow_calc/1(est_airflow) -> fuel_calc/1(est_airflow)
  sensors/1 -> control_logic/1(es_i), Bus Selector1/1
  control_logic/3(fuel_mode) -> airflow_calc/3(fuel_mode), fuel_calc/3(fuel_mode)
  control_logic/1(es_o) -> airflow_calc/1(sensors)
  control_logic/2(" O2_normal") -> airflow_calc/2(O2_normal)
  airflow_calc/2(fb_correction) -> fuel_calc/2(fb_correction)
  Bus Selector1/1 -> validate_sample_time/1(In1)  "<speed>"
